simulink model "DVVMPTC_motor"  (R2021a)
settings: Solver=VariableStepAuto  StartTime=0.0  StopTime=10.0  RelTol=1e-3
libraries: powerlib_extras x3, spsDCVoltageSourceLib x2, spsPermanentMagnetSynchronousMachineLib x2, spsUniversalBridgeLib x2, spsVoltageMeasurementLib x2, spspowerguiLib x2, pid_lib x1, simulink x1
settings Model: Creator=86188  LastModifiedBy=86188

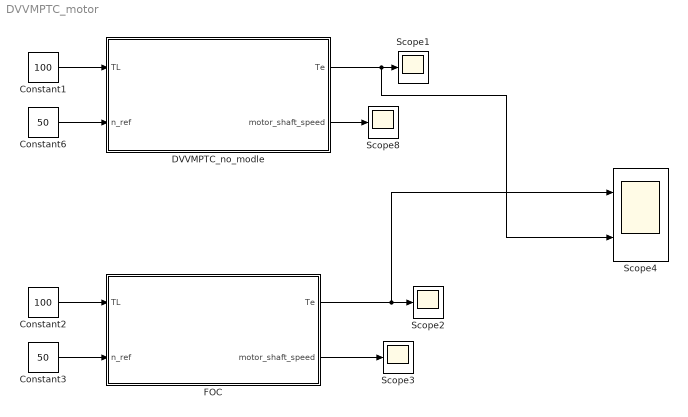
== system DVVMPTC_motor ==
  Constant1 : Constant  Value=100
  Constant2 : Constant  Value=100
  Constant3 : Constant  Value=50
  Constant6 : Constant  Value=50
  DVVMPTC_no_modle : Subsystem
  FOC : Subsystem
  Scope{1..3,8} (4 alike) : Scope
  Scope4 : Scope  NumInputPorts=2
  wires:
  DVVMPTC_no_modle/2(motor_shaft_speed) -> Scope8/1
  Constant1/1 -> DVVMPTC_no_modle/1(TL)
  Constant6/1 -> DVVMPTC_no_modle/2(n_ref)
  DVVMPTC_no_modle/1(Te) -> Scope4/2, Scope1/1
  Constant2/1 -> FOC/1(TL)
  Constant3/1 -> FOC/2(n_ref)
  FOC/1(Te) -> Scope4/1, Scope2/1
  FOC/2(motor_shaft_speed) -> Scope3/1

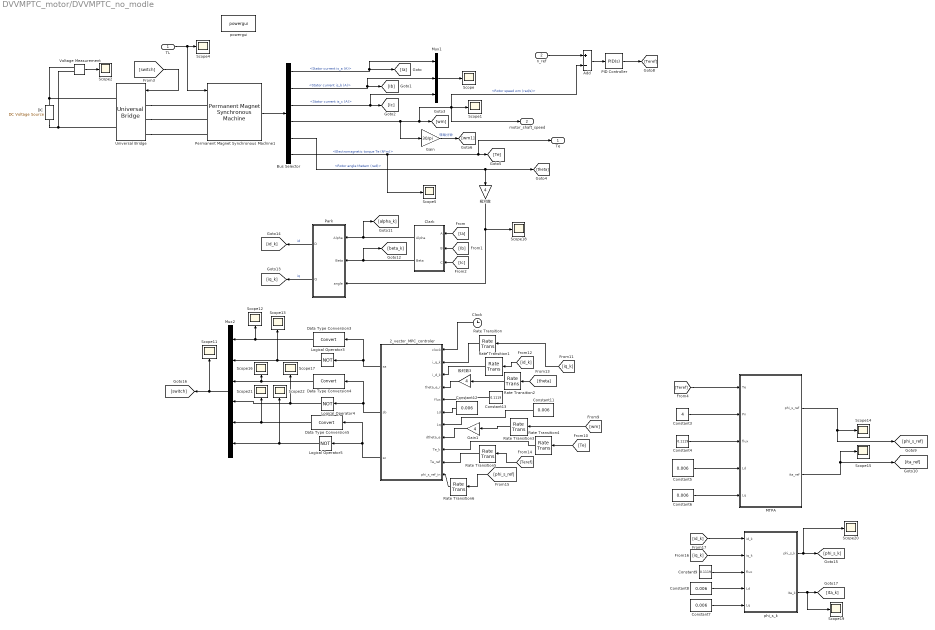
== system DVVMPTC_motor/DVVMPTC_no_modle ==
  TL : Inport
  n_ref : Inport  Port=2
  2_vector_MPC_controler : MATLAB Function  TreatAsAtomicUnit=on  SystemSampleTime=1e-5
  Add : Sum  Inputs=+-
  Bus Selector : BusSelector  OutputSignals=Stator current is_a (A),Stator current is_b (A),Stator current is_c (A),Rotor speed wm (rad/s),Rotor angle thetam (rad),Electromagnetic torque Te (N*m)
  Clark : Subsystem
  Clock : Clock
  Constant{5..8,11..12} (6 alike) : Constant  Value=0.006
  Constant13 : Constant  Value=0.1119
  Constant3 : Constant  Value=4
  Constant4 : Constant  Value=0.1119
  Constant9 : Constant  Value=0.1119
  DC : spsDCVoltageSourceLib/DC Voltage Source  Amplitude=400  Measurements=None
  Data Type Conversion3 : DataTypeConversion
  Data Type Conversion4 : DataTypeConversion
  Data Type Conversion5 : DataTypeConversion
  Gain : Gain  Gain=30/pi
  Gain1 : Gain  Gain=4
  Logical Operator3 : Logic  Operator=NOT  AllPortsSameDT=off  OutDataTypeStr=boolean
  Logical Operator4 : Logic  Operator=NOT  AllPortsSameDT=off  OutDataTypeStr=boolean
  Logical Operator5 : Logic  Operator=NOT  AllPortsSameDT=off  OutDataTypeStr=boolean
  MTPA : MATLAB Function  TreatAsAtomicUnit=on
  Mux1 : Mux  Inputs=3
  Mux2 : Mux  Inputs=6
  PID Controller : pid_lib/PID Controller  Controller=PID  Form=Parallel  TimeDomain=Continuous-time  UseExternalTs=off  SampleTime=-1  IntegratorMethod=Forward Euler  FilterMethod=Forward Euler  ControllerParametersSource=internal  P=5  I=1  D=0  UseFilter=on  N=100  TunerSelectOption=Transfer Function Based (PID Tuner App)  InitialConditionSource=internal  InitialConditionForIntegrator=0  InitialConditionForFilter=0  DifferentiatorICPrevScaledInput=0  ExternalReset=none  TrackingMode=off  Kt=1  LimitOutput=off  SatLimitsSource=internal  UpperSaturationLimit=inf  LowerSaturationLimit=-inf  LinearizeAsGain=on  AntiWindupMode=none  Kb=1  POutMin=[]  POutMax=[]  IOutMin=[]  IOutMax=[]  DOutMin=[]  DOutMax=[]  NOutMin=[]  NOutMax=[]  SumOutMin=[]  SumOutMax=[]  SaturationOutMin=[]  SaturationOutMax=[]  PParamMin=[]  PParamMax=[]  IParamMin=[]  IParamMax=[]  DParamMin=[]  DParamMax=[]  NParamMin=[]  NParamMax=[]  KbParamMin=[]  KbParamMax=[]  KtParamMin=[]  KtParamMax=[]  KbOutMin=[]  KbOutMax=[]  KtOutMin=[]  KtOutMax=[]  IntegratorOutMin=[]  IntegratorOutMax=[]  FilterOutMin=[]  FilterOutMax=[]  SumI1OutMin=[]  SumI1OutMax=[]  SumI2OutMin=[]  SumI2OutMax=[]  SumI3OutMin=[]  SumI3OutMax=[]  SumI4OutMin=[]  SumI4OutMax=[]  SumDOutMin=[]  SumDOutMax=[]  DifferentiatorOutMin=[]  DifferentiatorOutMax=[]  FilterDiffOutCoefMin=[]  FilterDiffOutCoefMax=[]  ReciprocalOutMin=[]  ReciprocalOutMax=[]  SumDenOutMin=[]  SumDenOutMax=[]  SumNumOutMin=[]  SumNumOutMax=[]  DivideOutMin=[]  DivideOutMax=[]  UdiffTsProdOutMin=[]  UdiffTsProdOutMax=[]  NTsProdOutMin=[]  NTsProdOutMax=[]  UintegralTsProdOutMin=[]  UintegralTsProdOutMax=[]  UngainTsProdOutMin=[]  UngainTsProdOutMax=[]  IntegratorContinuousStateAttributes=''  IntegratorStateMustResolveToSignalObject=off  IntegratorRTWStateStorageClass=Auto  FilterContinuousStateAttributes=''  FilterStateMustResolveToSignalObject=off  FilterRTWStateStorageClass=Auto  ParallelPVariant=InternalParameters  IdealPVariant=Disabled  IVariant=InternalParameters  DVariant=InternalParameters  IntegratorVariant=Continuous  SatVariant=Disabled  AWVariant=Passthrough  PCopyVariant=Disabled  TRVariant=Disabled  FdbkBlocksVariant=Forward  IdealPFdbkVariant=Disabled  SatFdbkVariant=Disabled  DerivativeFilterVariant=ContFilter  NVariant=InternalParameters  NCopyVariant=Disabled  FilterICVariant=InternalICsFilter  IntegratorICVariant=InternalICs  ExternalResetVariant=Disabled  TRSumVariant=Passthrough  SumFdbkVariant=Disabled  SumVariant=Sum_PID  TsampFilterVariant=InternalTs  TsampNgainVariant=Passthrough  TsampIntegralVariant=Passthrough  ExternalSaturationOutDataTypeStr=Inherit: Same as second input
  Park : Subsystem
  Permanent Magnet Synchronous Machine1 : spsPermanentMagnetSynchronousMachineLib/Permanent Magnet Synchronous Machine  NbPhases=3  FluxDistribution=Sinusoidal  RotorType=Salient-pole  MechanicalLoad=Torque Tm  PresetModel=No  ShowDetailedParameters=on  MeasurementBus=off  Resistance=0.11  Inductance=8.5e-3  dqInductances=[0.006 0.006]  La=0.000835  MachineConstant=Flux linkage established by magnets (V.s)  Flux=0.1119  VoltageCst=81.1857  TorqueCst=0.6714  Flat=120  Mechanical=[0.04 0.0002024 4 0]  PolePairs=4  InitialConditions=[0,0, 0,0]  InitialConditions5ph=[0 0 0 0 0 0]  RefAngle=Aligned with phase A axis (original Park)  IterativeDiscreteModel=Trapezoidal non iterative  TsBlock=-1  TsPowergui=0
  Rate Transition : RateTransition  OutPortSampleTime=1e-5
  Rate Transition1 : RateTransition  OutPortSampleTime=1e-5
  Rate Transition2 : RateTransition  OutPortSampleTime=1e-5
  Rate Transition{3..6} (4 alike) : RateTransition  OutPortSampleTime=1e-4
  Scope{,1..2,4..5,11..22} (17 alike) : Scope
  Universal Bridge : spsUniversalBridgeLib/Universal Bridge  Arms=3  SnubberResistance=1e5  SnubberCapacitance=inf  Device=IGBT / Diodes  Ron=1e-3  Lon=0  ForwardVoltages="[  0  0  ]"  ForwardVoltage=0  GTOparameters=[ 10e-6 , 20e-6 ]  IGBTparameters=[ 1e-6 , 2e-6 ]  Measurements=None  Measurements_2=None  converterType=Rectifier
  Voltage Measurement : spsVoltageMeasurementLib/Voltage Measurement  PhasorSimulation=off  OutputType=Complex  PSBequivalent=0
  phi_s_k : MATLAB Function  TreatAsAtomicUnit=on
  powergui : spspowerguiLib/powergui  Priority=1  SimulationMode=Discrete  SampleTime=1e-6  frequency=60  Iterations=50  frequencyindice=0  Pbase=100e6  ErrMax=1e-4  UnitsV=kV  UnitsW=MW  buscounter=0  FunctionMessages=off  echomessages=off  EnableUseOfTLC=off  CurrentSourceSwitches=off  DisableSnubberDevices=off  DisableRonSwitches=off  DisableVfSwitches=off  DisplayEquations=off  AutomaticDiscreteSolvers=off  SolverType=Tustin/Backward Euler (TBE)  Interpol=off  ExternalGateDelay=off  methode=off  Ts=100  x0status=blocks  SPID=on  SwTol=0  HookPort=off  NonlinearTolerance=1e-4  nMaxIteration=100  ContinueOnMaxIteration=off  RestoreLinks=warning  ResistiveCurrentMeasurement=off  Frange=[0:2:500]  Ylog=off  Xlog=on  ShowGrid=off  save=off  variable=ZData  structure=0  ZoomFFT=off  StartTime=0.0  cycles=1  DisplayStyle=1  fundamental=60  FreqAxis=off  MaxFrequency=1000  frequencyindicesteady=1  RmsSteady=1  display=off
  极对数 : Gain  Gain=4
  极对数3 : Gain  Gain=4
  Te : Outport
  motor_shaft_speed : Outport  Port=2
  wires:
  TL/1 -> Scope4/1, Permanent Magnet Synchronous Machine1/1
  Rate Transition6/1 -> 2_vector_MPC_controler/11(phi_s_ref_in)
  Rate Transition5/1 -> 2_vector_MPC_controler/10(Te_ref)
  Rate Transition4/1 -> 2_vector_MPC_controler/9(Te_k)
  Rate Transition3/1 -> Gain1/1
  Rate Transition2/1 -> 极对数3/1
  Rate Transition1/1 -> 2_vector_MPC_controler/3(i_d_k)
  Rate Transition/1 -> 2_vector_MPC_controler/2(i_q_k)
  phi_s_k/2(ita_k) -> [ita_k], Scope19/1
  极对数3/1 -> 2_vector_MPC_controler/4(theta_e_r)
  Mux2/1 -> [switch], Scope11/1
  Logical Operator5/1 -> Scope22/1, Mux2/6
  Data Type Conversion5/1 -> Scope21/1, Mux2/5
  Logical Operator4/1 -> Scope17/1, Mux2/4
  Data Type Conversion4/1 -> Scope16/1, Mux2/3
  Logical Operator3/1 -> Scope13/1, Mux2/2
  Data Type Conversion3/1 -> Scope12/1, Mux2/1
  2_vector_MPC_controler/3(sc) -> Logical Operator5/1, Data Type Conversion5/1
  2_vector_MPC_controler/2(sb) -> Logical Operator4/1, Data Type Conversion4/1
  2_vector_MPC_controler/1(sa) -> Logical Operator3/1, Data Type Conversion3/1
  [id_k] -> phi_s_k/1(id_k)
  [iq_k] -> phi_s_k/2(iq_k)
  phi_s_k/1(phi_s_k) -> Scope20/1, [phi_s_k]
  Constant9/1 -> phi_s_k/3(flux)
  Constant8/1 -> phi_s_k/4(Ld)
  Constant7/1 -> phi_s_k/5(Lq)
  MTPA/1(phi_s_ref) -> Scope14/1, [phi_s_ref]
  MTPA/2(ita_ref) -> [ita_ref], Scope15/1
  Constant6/1 -> MTPA/5(Lq)
  Constant5/1 -> MTPA/4(Ld)
  Constant4/1 -> MTPA/3(flux)
  Constant3/1 -> MTPA/2(Pn)
  [Teref] -> MTPA/1(Te)
  Clock/1 -> 2_vector_MPC_controler/1(clock)
  Permanent Magnet Synchronous Machine1/1 -> Bus Selector/1
  Bus Selector/1 -> Mux1/1, [Ia]  "<Stator current is_a (A)>"
  Bus Selector/2 -> Mux1/2, [Ib]  "<Stator current is_b (A)>"
  Bus Selector/3 -> Mux1/3, [Ic]  "<Stator current is_c (A)>"
  Bus Selector/4 -> Gain/1, motor_shaft_speed/1, Add/2, Scope1/1, [wm]  "<Rotor speed wm (rad/s)>"
  Bus Selector/5 -> 极对数/1, [theta]  "<Rotor angle thetam (rad)>"
  Bus Selector/6 -> [Te], Te/1, Scope5/1  "<Electromagnetic torque Te (N*m)>"
  Gain/1 -> [wm1]  "转每分钟"
  Clark/1(Alpha) -> Park/1(Alpha), [alpha_k]
  Clark/2(Beta) -> [beta_k], Park/2(Beta)
  [Ia] -> Clark/1(A)
  [Ib] -> Clark/2(B)
  [Ic] -> Clark/3(C)
  极对数/1 -> Park/3(angle), Scope18/1
  Park/1(D) -> [id_k]  "id"
  Park/2(Q) -> [iq_k]  "iq"
  [switch] -> Universal Bridge/1
  Mux1/1 -> Scope/1
  Gain1/1 -> 2_vector_MPC_controler/8(dtheta_e)
  Constant12/1 -> 2_vector_MPC_controler/6(Ld)
  Constant11/1 -> 2_vector_MPC_controler/7(Lq)
  Constant13/1 -> 2_vector_MPC_controler/5(flux)
  [Teref] -> Rate Transition5/1
  [phi_s_ref] -> Rate Transition6/1
  [iq_k] -> Rate Transition/1
  [id_k] -> Rate Transition1/1
  [theta] -> Rate Transition2/1
  [wm] -> Rate Transition3/1
  [Te] -> Rate Transition4/1
  n_ref/1 -> Add/1
  Voltage Measurement/1 -> Scope2/1
  PID Controller/1 -> [Teref]
  Add/1 -> PID Controller/1
  connections:
  Universal Bridge/LConn2 -- Permanent Magnet Synchronous Machine1/LConn2
  Universal Bridge/LConn3 -- Permanent Magnet Synchronous Machine1/LConn3
  DC/RConn1 -- Voltage Measurement/LConn1 -- Universal Bridge/RConn1
  DC/LConn1 -- Voltage Measurement/LConn2 -- Universal Bridge/RConn2
  Universal Bridge/LConn1 -- Permanent Magnet Synchronous Machine1/LConn1

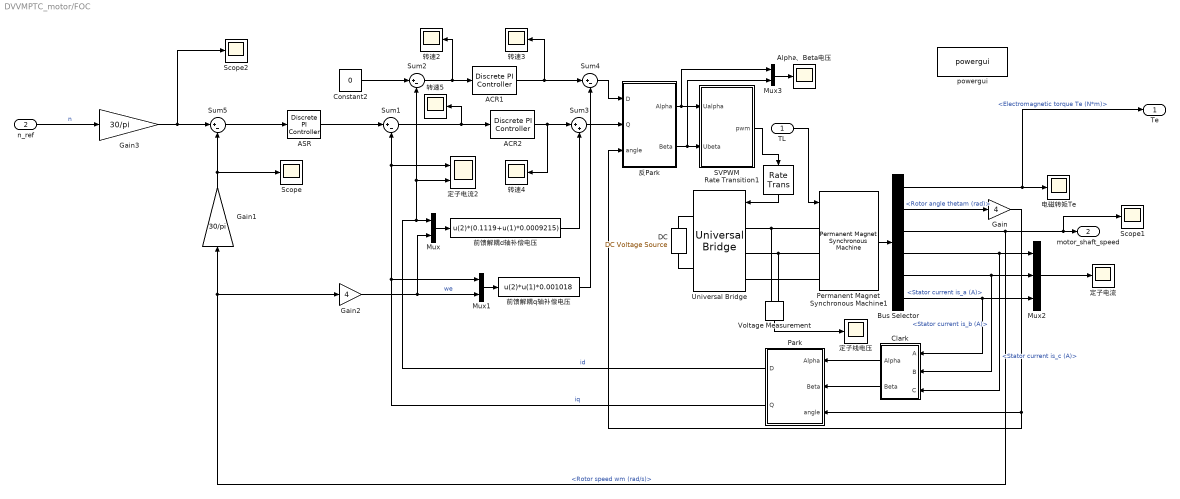
== system DVVMPTC_motor/FOC ==
  TL : Inport
  n_ref : Inport  Port=2
  ACR1 : powerlib_extras/Discrete  Control Blocks/Discrete PI Controller  Kp=4  Ki=80  Par_Limits=[760*0.9*sqrt(1/3) -760*0.9*sqrt(1/3)]  Init=0  Ts=1e-6
  ACR2 : powerlib_extras/Discrete  Control Blocks/Discrete PI Controller  Kp=4  Ki=80  Par_Limits=[760*0.9*sqrt(1/3) -760*0.9*sqrt(1/3)]  Init=0  Ts=1e-6
  ASR : powerlib_extras/Discrete  Control Blocks/Discrete PI Controller  Kp=0.8  Ki=10  Par_Limits=[1000 -1000]  Init=0  Ts=1e-6
  Alpha、Beta电压 : Scope
  Bus Selector : BusSelector  OutputSignals=Electromagnetic torque Te (N*m),Rotor angle thetam (rad),Rotor speed wm (rad/s),Stator current is_c (A),Stator current is_b (A),Stator current is_a (A)
  Clark : Subsystem
  Constant2 : Constant  Value=0
  DC : spsDCVoltageSourceLib/DC Voltage Source  Amplitude=560  Measurements=None
  Gain : Gain  Gain=4
  Gain1 : Gain  Gain=30/pi
  Gain2 : Gain  Gain=4
  Gain3 : Gain  Gain=30/pi
  Mux : Mux  Inputs=2
  Mux1 : Mux  Inputs=2
  Mux2 : Mux  Inputs=3
  Mux3 : Mux  Inputs=2
  Park : Subsystem
  Permanent Magnet Synchronous Machine1 : spsPermanentMagnetSynchronousMachineLib/Permanent Magnet Synchronous Machine  NbPhases=3  FluxDistribution=Sinusoidal  RotorType=Salient-pole  MechanicalLoad=Torque Tm  PresetModel=No  ShowDetailedParameters=on  MeasurementBus=off  Resistance=0.11  Inductance=8.5e-3  dqInductances=[0.006 0.006]  La=0.000835  MachineConstant=Flux linkage established by magnets (V.s)  Flux=0.1119  VoltageCst=81.1857  TorqueCst=0.6714  Flat=120  Mechanical=[0.04 0.0002024 4 0]  PolePairs=4  InitialConditions=[0,0, 0,0]  InitialConditions5ph=[0 0 0 0 0 0]  RefAngle=Aligned with phase A axis (original Park)  IterativeDiscreteModel=Trapezoidal non iterative  TsBlock=-1  TsPowergui=0
  Rate Transition1 : RateTransition  OutPortSampleTime=1e-5
  SVPWM : Subsystem
  Scope : Scope
  Scope1 : Scope
  Scope2 : Scope
  Sum{1..2,4..5} (4 alike) : Sum  Inputs=|+-
  Sum3 : Sum  Inputs=|++
  Universal Bridge : spsUniversalBridgeLib/Universal Bridge  Arms=3  SnubberResistance=1e5  SnubberCapacitance=inf  Device=IGBT / Diodes  Ron=1e-3  Lon=0  ForwardVoltages="[  0  0  ]"  ForwardVoltage=0  GTOparameters=[ 10e-6 , 20e-6 ]  IGBTparameters=[ 1e-6 , 2e-6 ]  Measurements=None  Measurements_2=None  converterType=Rectifier
  Voltage Measurement : spsVoltageMeasurementLib/Voltage Measurement  PhasorSimulation=off  OutputType=Complex  PSBequivalent=0
  powergui : spspowerguiLib/powergui  Priority=1  SimulationMode=Discrete  SampleTime=1e-6  frequency=60  Iterations=50  frequencyindice=0  Pbase=100e6  ErrMax=1e-4  UnitsV=kV  UnitsW=MW  buscounter=0  FunctionMessages=off  echomessages=off  EnableUseOfTLC=off  CurrentSourceSwitches=off  DisableSnubberDevices=off  DisableRonSwitches=off  DisableVfSwitches=off  DisplayEquations=off  AutomaticDiscreteSolvers=off  SolverType=Tustin  Interpol=off  ExternalGateDelay=off  methode=off  Ts=0  x0status=blocks  SPID=off  SwTol=0  HookPort=off  NonlinearTolerance=1e-4  nMaxIteration=100  ContinueOnMaxIteration=off  RestoreLinks=warning  ResistiveCurrentMeasurement=off  Frange=[0:2:500]  Ylog=off  Xlog=on  ShowGrid=off  save=off  variable=ZData  structure=ScopeData7  ZoomFFT=on  StartTime=2.5  cycles=3  DisplayStyle=1  fundamental=60  FreqAxis=off  MaxFrequency=2000  frequencyindicesteady=1  RmsSteady=1  display=off
  前馈解耦d轴补偿电压 : Fcn  Expr=u(2)*(0.1119+u(1)*0.0009215)
  前馈解耦q轴补偿电压 : Fcn  Expr=u(2)*u(1)*0.001018
  反Park : Subsystem
  定子电流 : Scope
  定子电流2 : Scope  NumInputPorts=2
  定子线电压 : Scope
  电磁转矩Te : Scope
  转速{2..5} (4 alike) : Scope
  Te : Outport
  motor_shaft_speed : Outport  Port=2
  wires:
  Gain3/1 -> Sum5/1, Scope2/1
  Gain1/1 -> Scope/1, Sum5/2
  ASR/1 -> Sum1/1
  Voltage Measurement/1 -> 定子线电压/1
  前馈解耦q轴补偿电压/1 -> Sum4/2
  Sum2/1 -> ACR1/1, 转速2/1
  Mux2/1 -> 定子电流/1
  Bus Selector/6 -> Clark/1(A), Mux2/3  "<Stator current is_a (A)>"
  Sum5/1 -> ASR/1
  Clark/1(Alpha) -> Park/1(Alpha)
  Permanent Magnet Synchronous Machine1/1 -> Bus Selector/1
  Park/2(Q) -> Sum1/2, 定子电流2/1, Mux1/1  "iq"
  Clark/2(Beta) -> Park/2(Beta)
  Sum1/1 -> ACR2/1, 转速5/1
  Mux3/1 -> Alpha、Beta电压/1
  反Park/1(Alpha) -> SVPWM/1(Ualpha), Mux3/1
  Bus Selector/3 -> motor_shaft_speed/1, Scope1/1, Gain1/1, Gain2/1  "<Rotor speed wm (rad/s)>"
  Mux/1 -> 前馈解耦d轴补偿电压/1
  反Park/2(Beta) -> SVPWM/2(Ubeta), Mux3/2
  Sum3/1 -> 反Park/2(Q)
  Park/1(D) -> Mux/1, Sum2/2, 定子电流2/2  "id"
  Bus Selector/1 -> 电磁转矩Te/1, Te/1  "<Electromagnetic torque Te (N*m)>"
  Bus Selector/5 -> Clark/2(B), Mux2/2  "<Stator current is_b (A)>"
  Bus Selector/2 -> Gain/1  "<Rotor angle thetam (rad)>"
  n_ref/1 -> Gain3/1  "n"
  前馈解耦d轴补偿电压/1 -> Sum3/2
  ACR2/1 -> Sum3/1, 转速4/1
  Sum4/1 -> 反Park/1(D)
  SVPWM/1(pwm) -> Rate Transition1/1
  Mux1/1 -> 前馈解耦q轴补偿电压/1
  Gain2/1 -> Mux/2, Mux1/2  "we"
  Gain/1 -> Park/3(angle), 反Park/3(angle)
  Constant2/1 -> Sum2/1
  Bus Selector/4 -> Clark/3(C), Mux2/1  "<Stator current is_c (A)>"
  ACR1/1 -> Sum4/1, 转速3/1
  TL/1 -> Permanent Magnet Synchronous Machine1/1
  Rate Transition1/1 -> Universal Bridge/1
  connections:
  Voltage Measurement/LConn1 -- Permanent Magnet Synchronous Machine1/LConn1 -- Universal Bridge/LConn1
  Voltage Measurement/LConn2 -- Permanent Magnet Synchronous Machine1/LConn2 -- Universal Bridge/LConn2
  DC/RConn1 -- Universal Bridge/RConn1
  Permanent Magnet Synchronous Machine1/LConn3 -- Universal Bridge/LConn3
  DC/LConn1 -- Universal Bridge/RConn2

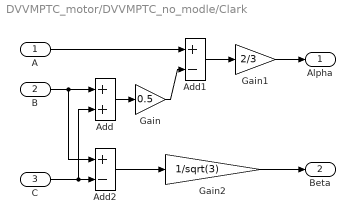
== system DVVMPTC_motor/DVVMPTC_no_modle/Clark ==
  A : Inport
  B : Inport  Port=2
  C : Inport  Port=3
  Add : Sum
  Add1 : Sum  Inputs=+-
  Add2 : Sum  Inputs=+-
  Gain : Gain  Gain=0.5
  Gain1 : Gain  Gain=2/3
  Gain2 : Gain  Gain=1/sqrt(3)
  Alpha : Outport
  Beta : Outport  Port=2
  wires:
  B/1 -> Add2/1, Add/1
  C/1 -> Add/2, Add2/2
  Add/1 -> Gain/1
  A/1 -> Add1/1
  Gain/1 -> Add1/2
  Add1/1 -> Gain1/1
  Gain1/1 -> Alpha/1
  Add2/1 -> Gain2/1
  Gain2/1 -> Beta/1

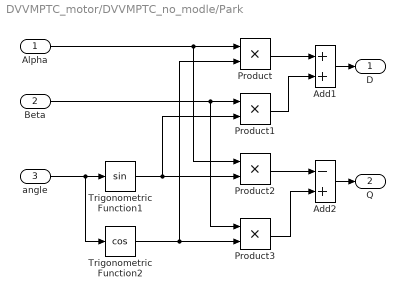
== system DVVMPTC_motor/DVVMPTC_no_modle/Park ==
  Alpha : Inport
  Beta : Inport  Port=2
  angle : Inport  Port=3
  Add1 : Sum
  Add2 : Sum  Inputs=-+
  Product{,1..3} (4 alike) : Product
  Trigonometric Function1 : Trigonometry
  Trigonometric Function2 : Trigonometry  Operator=cos
  D : Outport
  Q : Outport  Port=2
  wires:
  Add2/1 -> Q/1
  Product3/1 -> Add2/2
  Product2/1 -> Add2/1
  Add1/1 -> D/1
  Product1/1 -> Add1/2
  Product/1 -> Add1/1
  Trigonometric Function1/1 -> Product2/2, Product1/2
  Beta/1 -> Product3/1, Product1/1
  Trigonometric Function2/1 -> Product3/2, Product/2
  Alpha/1 -> Product2/1, Product/1
  angle/1 -> Trigonometric Function1/1, Trigonometric Function2/1

== system DVVMPTC_motor/FOC/Clark ==
  A : Inport
  B : Inport  Port=2
  C : Inport  Port=3
  Add : Sum
  Add1 : Sum  Inputs=+-
  Add2 : Sum  Inputs=+-
  Gain : Gain  Gain=0.5
  Gain1 : Gain  Gain=2/3
  Gain2 : Gain  Gain=1/sqrt(3)
  Alpha : Outport
  Beta : Outport  Port=2
  wires:
  Gain2/1 -> Beta/1
  Add2/1 -> Gain2/1
  Gain1/1 -> Alpha/1
  Add1/1 -> Gain1/1
  Gain/1 -> Add1/2
  A/1 -> Add1/1
  Add/1 -> Gain/1
  C/1 -> Add2/2, Add/2
  B/1 -> Add/1, Add2/1

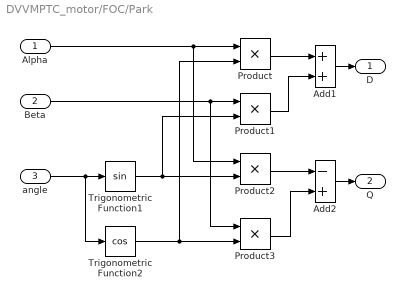
== system DVVMPTC_motor/FOC/Park ==
  Alpha : Inport
  Beta : Inport  Port=2
  angle : Inport  Port=3
  Add1 : Sum
  Add2 : Sum  Inputs=-+
  Product{,1..3} (4 alike) : Product
  Trigonometric Function1 : Trigonometry
  Trigonometric Function2 : Trigonometry  Operator=cos
  D : Outport
  Q : Outport  Port=2
  wires:
  angle/1 -> Trigonometric Function2/1, Trigonometric Function1/1
  Alpha/1 -> Product/1, Product2/1
  Trigonometric Function2/1 -> Product/2, Product3/2
  Beta/1 -> Product1/1, Product3/1
  Trigonometric Function1/1 -> Product1/2, Product2/2
  Product/1 -> Add1/1
  Product1/1 -> Add1/2
  Add1/1 -> D/1
  Product2/1 -> Add2/1
  Product3/1 -> Add2/2
  Add2/1 -> Q/1

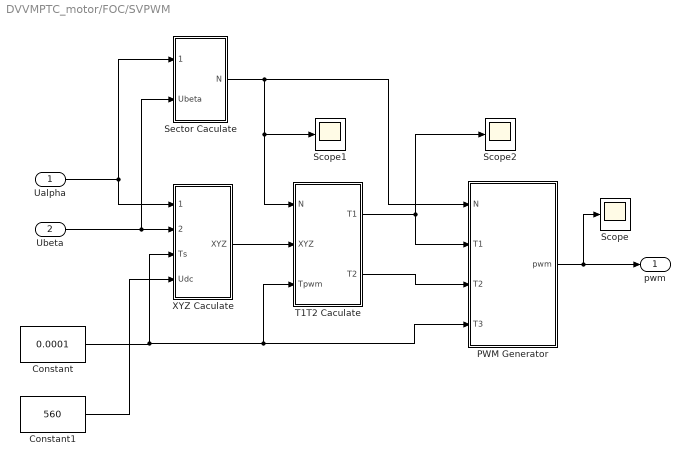
== system DVVMPTC_motor/FOC/SVPWM ==
  Ualpha : Inport
  Ubeta : Inport  Port=2
  Constant : Constant  Value=0.0001
  Constant1 : Constant  Value=560
  PWM Generator : Subsystem
  Scope : Scope
  Scope1 : Scope
  Scope2 : Scope
  Sector Caculate : Subsystem
  T1T2 Caculate : Subsystem
  XYZ Caculate : Subsystem
  pwm : Outport
  wires:
  PWM Generator/1(pwm) -> Scope/1, pwm/1
  T1T2 Caculate/2(T2) -> PWM Generator/3(T2)
  T1T2 Caculate/1("T1 ") -> Scope2/1, PWM Generator/2(T1)
  Sector Caculate/1(N) -> PWM Generator/1(N), T1T2 Caculate/1(N), Scope1/1
  XYZ Caculate/1(XYZ) -> T1T2 Caculate/2(XYZ)
  Constant1/1 -> XYZ Caculate/4(Udc)
  Constant/1 -> XYZ Caculate/3(Ts), T1T2 Caculate/3(Tpwm), PWM Generator/4(T3)
  Ubeta/1 -> XYZ Caculate/2(Ubeta), Sector Caculate/2("Ubeta ")
  Ualpha/1 -> Sector Caculate/1(Ualpha), XYZ Caculate/1(Ualpha)

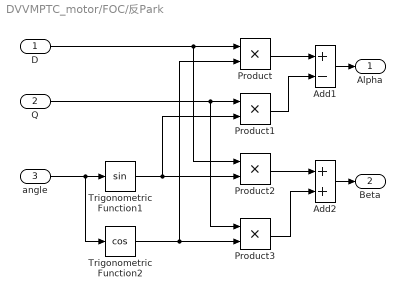
== system DVVMPTC_motor/FOC/反Park ==
  D : Inport
  Q : Inport  Port=2
  angle : Inport  Port=3
  Add1 : Sum  Inputs=+-
  Add2 : Sum
  Product{,1..3} (4 alike) : Product
  Trigonometric Function1 : Trigonometry
  Trigonometric Function2 : Trigonometry  Operator=cos
  Alpha : Outport
  Beta : Outport  Port=2
  wires:
  Add2/1 -> Beta/1
  Product3/1 -> Add2/2
  Product2/1 -> Add2/1
  Add1/1 -> Alpha/1
  Product1/1 -> Add1/2
  Product/1 -> Add1/1
  Trigonometric Function1/1 -> Product2/2, Product1/2
  Q/1 -> Product3/1, Product1/1
  Trigonometric Function2/1 -> Product3/2, Product/2
  D/1 -> Product2/1, Product/1
  angle/1 -> Trigonometric Function1/1, Trigonometric Function2/1

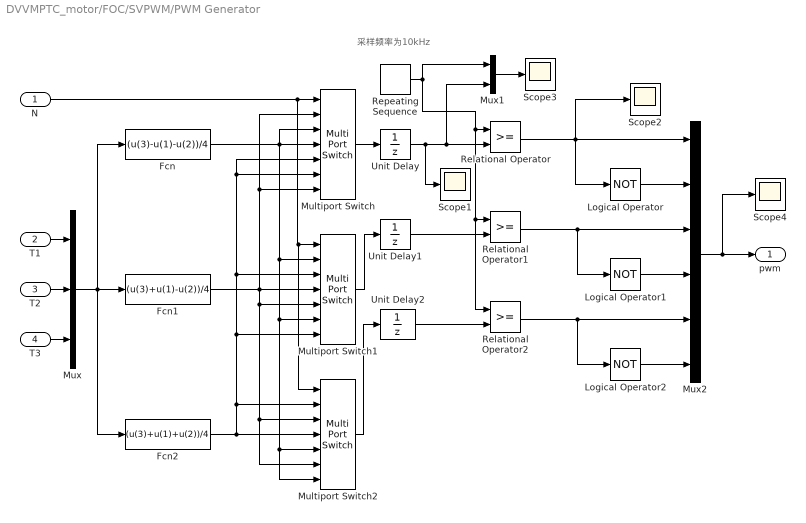
== system DVVMPTC_motor/FOC/SVPWM/PWM Generator ==
  note: 采样频率为10kHz
  N : Inport
  T1 : Inport  Port=2
  T2 : Inport  Port=3
  T3 : Inport  Port=4
  Fcn : Fcn  Expr=(u(3)-u(1)-u(2))/4
  Fcn1 : Fcn  Expr=(u(3)+u(1)-u(2))/4
  Fcn2 : Fcn  Expr=(u(3)+u(1)+u(2))/4
  Logical Operator : Logic  Operator=NOT  AllPortsSameDT=off  OutDataTypeStr=boolean
  Logical Operator1 : Logic  Operator=NOT  AllPortsSameDT=off  OutDataTypeStr=boolean
  Logical Operator2 : Logic  Operator=NOT  AllPortsSameDT=off  OutDataTypeStr=boolean
  Multiport Switch : MultiPortSwitch  Inputs=6  DiagnosticForDefault=None
  Multiport Switch1 : MultiPortSwitch  Inputs=6  DiagnosticForDefault=None
  Multiport Switch2 : MultiPortSwitch  Inputs=6  DiagnosticForDefault=None
  Mux : Mux  Inputs=3
  Mux1 : Mux  Inputs=2
  Mux2 : Mux  Inputs=6
  Relational Operator : RelationalOperator  OutDataTypeStr=boolean  RndMeth=Nearest
  Relational Operator1 : RelationalOperator  OutDataTypeStr=boolean  RndMeth=Nearest
  Relational Operator2 : RelationalOperator  OutDataTypeStr=boolean  RndMeth=Nearest
  Repeating Sequence : simulink/Sources/Repeating Sequence  rep_seq_t=[0 0.00005 0.0001]  rep_seq_y=[0 0.00005 0]
  Scope{1..4} (4 alike) : Scope
  Unit Delay : UnitDelay  SampleTime=0.0001  HasFrameUpgradeWarning=on
  Unit Delay1 : UnitDelay  SampleTime=0.0001  HasFrameUpgradeWarning=on
  Unit Delay2 : UnitDelay  SampleTime=0.0001  HasFrameUpgradeWarning=on
  pwm : Outport
  wires:
  Unit Delay2/1 -> Relational Operator2/2
  Unit Delay1/1 -> Relational Operator1/2
  Unit Delay/1 -> Scope1/1, Relational Operator/2, Mux1/2
  Mux1/1 -> Scope3/1
  Multiport Switch/1 -> Unit Delay/1
  Multiport Switch2/1 -> Unit Delay2/1
  Multiport Switch1/1 -> Unit Delay1/1
  Mux2/1 -> pwm/1, Scope4/1
  Logical Operator2/1 -> Mux2/6
  Logical Operator1/1 -> Mux2/4
  Logical Operator/1 -> Mux2/2
  Relational Operator2/1 -> Mux2/5, Logical Operator2/1
  Relational Operator1/1 -> Mux2/3, Logical Operator1/1
  Relational Operator/1 -> Mux2/1, Logical Operator/1, Scope2/1
  Repeating Sequence/1 -> Relational Operator/1, Relational Operator1/1, Relational Operator2/1, Mux1/1
  Fcn2/1 -> Multiport Switch/5, Multiport Switch/6, Multiport Switch1/3, Multiport Switch1/7, Multiport Switch2/2, Multiport Switch2/4
  Fcn1/1 -> Multiport Switch1/4, Multiport Switch1/5, Multiport Switch2/3, Multiport Switch2/6, Multiport Switch/2, Multiport Switch/7
  Fcn/1 -> Multiport Switch/3, Multiport Switch/4, Multiport Switch1/2, Multiport Switch1/6, Multiport Switch2/5, Multiport Switch2/7
  N/1 -> Multiport Switch/1, Multiport Switch1/1, Multiport Switch2/1
  Mux/1 -> Fcn2/1, Fcn1/1, Fcn/1
  T3/1 -> Mux/3
  T1/1 -> Mux/1
  T2/1 -> Mux/2

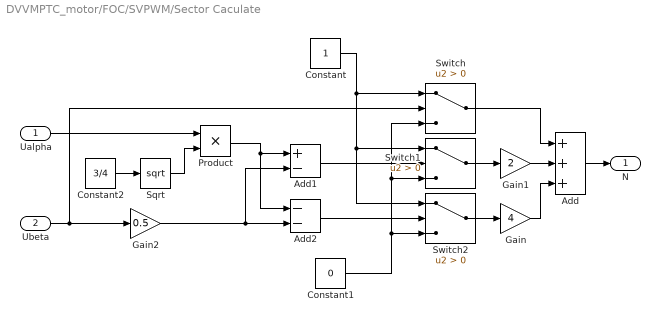
== system DVVMPTC_motor/FOC/SVPWM/Sector Caculate ==
  Ualpha : Inport
  "Ubeta " : Inport  Port=2
  Add : Sum  Inputs=+++
  Add1 : Sum  Inputs=+-
  Add2 : Sum  Inputs=--
  Constant : Constant
  Constant1 : Constant  Value=0
  Constant2 : Constant  Value=3/4
  Gain : Gain  Gain=4
  Gain1 : Gain  Gain=2
  Gain2 : Gain  Gain=0.5
  Product : Product
  Sqrt : Sqrt  SaturateOnIntegerOverflow=on
  Switch : Switch  Criteria=u2 > Threshold
  Switch1 : Switch  Criteria=u2 > Threshold
  Switch2 : Switch  Criteria=u2 > Threshold
  N : Outport
  wires:
  Gain2/1 -> Add2/2, Add1/2
  Product/1 -> Add1/1, Add2/1
  Sqrt/1 -> Product/2
  Constant2/1 -> Sqrt/1
  Switch/1 -> Add/1
  Switch1/1 -> Gain1/1
  Switch2/1 -> Gain/1
  Gain/1 -> Add/3
  Gain1/1 -> Add/2
  Add/1 -> N/1
  Constant1/1 -> Switch/3, Switch1/3, Switch2/3
  Constant/1 -> Switch2/1, Switch1/1, Switch/1
  Add2/1 -> Switch2/2
  Add1/1 -> Switch1/2
  "Ubeta "/1 -> Gain2/1, Switch/2
  Ualpha/1 -> Product/1

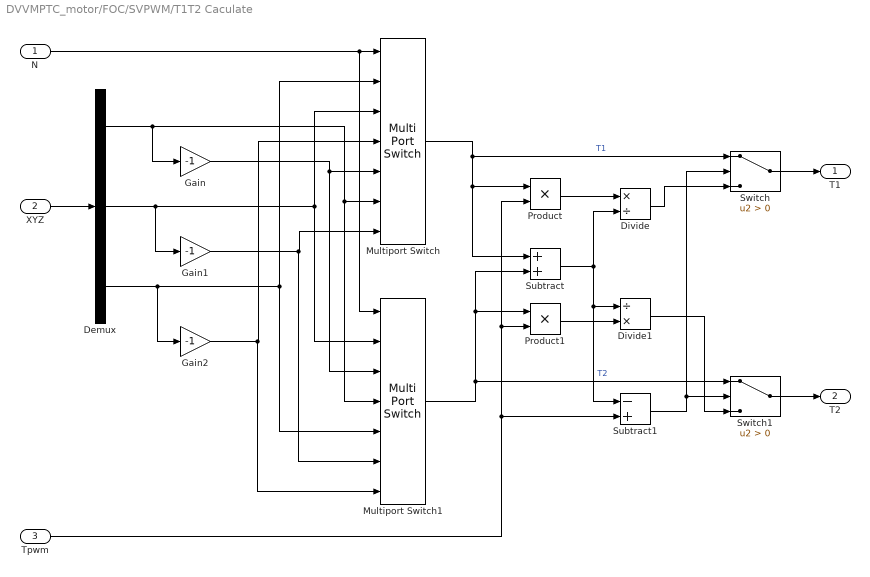
== system DVVMPTC_motor/FOC/SVPWM/T1T2 Caculate ==
  N : Inport
  XYZ : Inport  Port=2
  Tpwm : Inport  Port=3
  Demux : Demux  Outputs=3
  Divide : Product  Inputs=*/
  Divide1 : Product  Inputs=/*
  Gain : Gain  Gain=-1
  Gain1 : Gain  Gain=-1
  Gain2 : Gain  Gain=-1
  Multiport Switch : MultiPortSwitch  Inputs=6  DiagnosticForDefault=None
  Multiport Switch1 : MultiPortSwitch  Inputs=6  DiagnosticForDefault=None
  Product : Product
  Product1 : Product
  Subtract : Sum
  Subtract1 : Sum  Inputs=-+
  Switch : Switch  Criteria=u2 > Threshold
  Switch1 : Switch  Criteria=u2 > Threshold
  "T1 " : Outport
  T2 : Outport  Port=2
  wires:
  Product1/1 -> Divide1/2
  Subtract/1 -> Subtract1/1, Divide1/1, Divide/2
  Product/1 -> Divide/1
  Switch/1 -> "T1 "/1
  Switch1/1 -> T2/1
  Subtract1/1 -> Switch/2, Switch1/2
  Divide1/1 -> Switch1/3
  Divide/1 -> Switch/3
  Tpwm/1 -> Product1/2, Product/2, Subtract1/2
  Multiport Switch1/1 -> Switch1/1, Product1/1, Subtract/2  "T2"
  Multiport Switch/1 -> Subtract/1, Product/1, Switch/1  "T1"
  XYZ/1 -> Demux/1
  Gain2/1 -> Multiport Switch/4, Multiport Switch1/7
  Gain1/1 -> Multiport Switch/7, Multiport Switch1/6
  Gain/1 -> Multiport Switch1/3, Multiport Switch/5
  Demux/3 -> Multiport Switch/2, Multiport Switch1/5, Gain2/1
  Demux/2 -> Gain1/1, Multiport Switch1/2, Multiport Switch/3
  Demux/1 -> Gain/1, Multiport Switch/6, Multiport Switch1/4
  N/1 -> Multiport Switch/1, Multiport Switch1/1

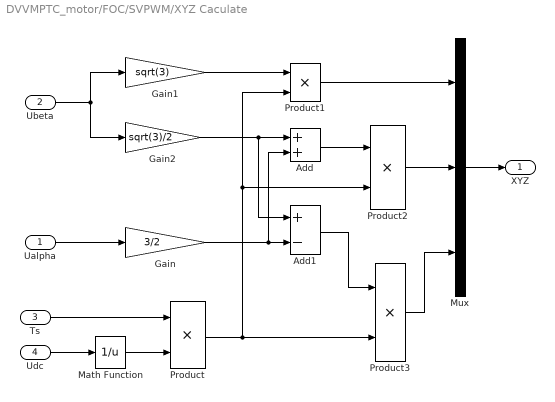
== system DVVMPTC_motor/FOC/SVPWM/XYZ Caculate ==
  Ualpha : Inport
  Ubeta : Inport  Port=2
  Ts : Inport  Port=3
  Udc : Inport  Port=4
  Add : Sum
  Add1 : Sum  Inputs=+-
  Gain : Gain  Gain=3/2
  Gain1 : Gain  Gain=sqrt(3)
  Gain2 : Gain  Gain=sqrt(3)/2
  Math Function : Math  Operator=reciprocal  SignedPower=on  SaturateOnIntegerOverflow=on
  Mux : Mux  Inputs=3
  Product{,1..3} (4 alike) : Product
  XYZ : Outport
  wires:
  Mux/1 -> XYZ/1
  Product2/1 -> Mux/2
  Add1/1 -> Product3/1
  Add/1 -> Product2/1
  Gain2/1 -> Add/1, Add1/1
  Gain/1 -> Add1/2, Add/2
  Product3/1 -> Mux/3
  Product/1 -> Product3/2, Product2/2, Product1/2
  Product1/1 -> Mux/1
  Gain1/1 -> Product1/1
  Math Function/1 -> Product/2
  Udc/1 -> Math Function/1
  Ts/1 -> Product/1
  Ubeta/1 -> Gain1/1, Gain2/1
  Ualpha/1 -> Gain/1

== matlab function DVVMPTC_motor/DVVMPTC_no_modle/2_vector_MPC_controler ==
  settings: updateMethod=DISCRETE
  data: clock input; i_q_k input; i_d_k input; theta_e_r input; sa output; sb output; sc output; flux input; Ld input; Lq input; dtheta_e input; Te_k input; Te_ref input; phi_s_ref_in input
function [sa, sb, sc] = fcn(clock, i_q_k, i_d_k, theta_e_r, flux, Ld, Lq, dtheta_e, Te_k, Te_ref, phi_s_ref_in)
    %% 0. 参数初始化
    Ts = 0.0001;     % 控制周期 100us
    vdc = 400;       % 母线电压
    Rs = 0.11;       % 定子电阻
    pn = 4;          % 极对数
    
    %% 1. 状态预测（一拍延时补偿） - 核心修复点
    % 论文公式 (5) 或 (6)。此处使用前向欧拉法预测 k+1 时刻的电流
    % 注意：此时假定 k 时刻施加的电压是上一个周期计算出的最优电压
    % 但在 Simulink 仿真中，通常需要将上个周期的 u_opt 反馈回来。
    % 如果没有反馈，可以用近似方法：假设当前电流已经包含了一部分过去的影响，
    % 但更标准的做法是预测。这里简化处理，基于当前电流和反电势预测下一刻的趋势。
    
    % 在实际 MPTC 中，必须利用 k 时刻的 u(k) 来预测 i(k+1)
    % 这里为了简化，我们至少要补偿旋转导致的相位角变化
    theta_e_k1 = theta_e_r + dtheta_e * Ts; 
    
    % 使用论文公式(5)进行电流预测 (需要上个周期的电压，这里暂用反电势模型近似补偿相位)
    % 严谨做法：Function 增加输入 u_alpha_old, u_beta_old
    % 这里采用论文中忽略电阻压降后的磁链预测公式(7)的简化逻辑：
    
    % 计算 k 时刻的磁链
    phi_d_k = Ld * i_d_k + flux;
    phi_q_k = Lq * i_q_k;
    
    % 预测 k+1 时刻的磁链 (基于旋转坐标系，假设稳态时 d/dt=0，主要变化由旋转引起)
    % 论文公式 (7) 的核心思想
    phi_d_k1 = phi_d_k + (dtheta_e * phi_q_k) * Ts; 
    phi_q_k1 = phi_q_k - (dtheta_e * phi_d_k) * Ts;
    
    % 更新预测后的电流 (用于后续计算)
    % i_d_k1 = (phi_d_k1 - flux) / Ld; % 如果是 IPMSM
    % i_q_k1 = phi_q_k1 / Lq;
    
    % 为了解决"掉落到负载转矩"的问题，必须修正用于计算参考电压的磁链值
    % 使用预测值代替测量值
    phi_d_calc = phi_d_k1;
    phi_q_calc = phi_q_k1;
    
    %% 2. 磁链参考值修正 - 核心修复点
    % 死拍控制要求非常严格，如果 Te_ref 很大，导致需要的 iq 很大，
    % 此时总磁链 sqrt(phid^2 + phiq^2) 必然增加。
    % 如果输入的 phi_s_ref 太小（例如只给 flux），方程无解，导致转矩上不去。
    % 这里根据 MTPA (id=0) 原则动态计算最小所需磁链
    
    % 基于 MTPA (id=0) 计算期望的 q 轴磁链
    expected_iq = Te_ref / (1.5 * pn * flux); 
    expected_phi_q = Lq * expected_iq;
    expected_phi_d = flux; % id=0 时
    
    % 计算物理上兼容的磁链参考值
    min_phi_s = sqrt(expected_phi_d^2 + expected_phi_q^2);
    
    % 如果输入的参考值小于物理限制，则覆盖它
    if phi_s_ref_in < min_phi_s
        phi_s_ref = min_phi_s;
    else
        phi_s_ref = phi_s_ref_in;
    end

    %% 3. DB-DTFC 计算参考电压 (基于预测的 k+1 状态计算 k+2 的需求)
    % 论文公式 (12) 和相关系数
    % X1 对应 d 轴电压方程中的耦合项
    X1 = phi_d_calc + dtheta_e * phi_q_calc * Ts;
    
    % B 对应 q 轴电压方程中的项 (包含转矩误差反馈)
    % 注意：这里用 Te_ref - Te_k，如果 Te_k 滞后，这里增益会很大。
    % 理想情况下应使用预测转矩 Te_k1，但使用 Te_k 在低速下尚可。
    B = ((2*Lq)/(3*pn*flux))*(Te_ref - Te_k) + (Rs*Ts*phi_q_calc)/Lq + dtheta_e*Ts*phi_d_calc;
    
    % 求解 d 轴电压 (二次方程)
    % (X1 + ud*Ts)^2 + (B)^2 = phi_s_ref^2
    % 展开：X1^2 + 2*X1*ud*Ts + ud^2*Ts^2 + B^2 = phi_s_ref^2
    % 整理为标准形式 a*x^2 + b*x + c = 0
    % a = Ts^2
    % b = 2*X1*Ts
    % c = X1^2 + B^2 - phi_s_ref^2
    
    % 你原本的代码逻辑似乎来源于论文的另一种推导，但这里直接用勾股定理推导更直观且等价
    % 你的代码 X2 计算有点复杂，这里简化逻辑以确保数值稳定
    
    term_c = X1^2 + B^2 - phi_s_ref^2;
    delta = (2*X1*Ts)^2 - 4 * (Ts^2) * term_c;
    
    if delta < 0
        delta = 0; % 强行有解，防止复数
    end
    
    % 求解 ud
    ud_sol1 = (-2*X1*Ts + sqrt(delta)) / (2*Ts^2);
    ud_sol2 = (-2*X1*Ts - sqrt(delta)) / (2*Ts^2);
    
    % 选择绝对值较小的电压矢量（能量最小原理）
    if abs(ud_sol1) < abs(ud_sol2)
        ud_ref = ud_sol1;
    else
        ud_ref = ud_sol2;
    end
    
    uq_ref = B / Ts;

    %% 4. 坐标变换 (dq -> alpha/beta)
    % 注意：必须使用 k+1 时刻的角度进行变换，因为电压是在 k+1 时刻发出的
    u_alpha_ref = cos(theta_e_k1)*ud_ref - sin(theta_e_k1)*uq_ref;
    u_beta_ref  = sin(theta_e_k1)*ud_ref + cos(theta_e_k1)*uq_ref;
    
    theta_u_ref = atan2(u_beta_ref, u_alpha_ref);
    if theta_u_ref < 0
        theta_u_ref = theta_u_ref + 2*pi;
    end

    %% 5. 第一扇区及矢量选择
    theta_norm_rel = theta_u_ref + pi/6; % 偏移30度以匹配扇区定义
    if theta_norm_rel > 2*pi
        theta_norm_rel = theta_norm_rel - 2*pi;
    end

    sector = floor(theta_norm_rel / (pi/3)) + 1;
    if sector > 6 
        sector = 1; % 修正 sector=7 的情况
    end
    
    % 电压矢量定义 (0-7)
    % 对应: V0, V1(100), V2(110), V3(010), V4(011), V5(001), V6(101), V7
    voltage_vectors = [
        0 0 0; % 0 (Index 1)
        1 0 0; % 1 (Index 2)
        1 1 0; % 2 (Index 3)
        0 1 0; % 3 (Index 4)
        0 1 1; % 4 (Index 5)
        0 0 1; % 5 (Index 6)
        1 0 1; % 6 (Index 7)
        1 1 1];% 7 (Index 8)

    first_vector_idx = sector + 1; 
    first_vector = voltage_vectors(first_vector_idx, :);

    %% 6. 第二矢量选择 (MPTC-II: 遍历相邻矢量)
    % 将 Alpha-Beta 坐标系下的 8 个基础电压矢量预先计算出来
    v_basic_alpha = zeros(8,1);
    v_basic_beta = zeros(8,1);
    const_k = 2/3 * vdc;
    for k = 1:8
        sa_t = voltage_vectors(k,1); sb_t = voltage_vectors(k,2); sc_t = voltage_vectors(k,3);
        u_an = vdc/3 * (2*sa_t - sb_t - sc_t);
        u_bn = vdc/3 * (2*sb_t - sa_t - sc_t);
        u_cn = vdc/3 * (2*sc_t - sa_t - sb_t); % 仅用于推导
        v_basic_alpha(k) = u_an;
        v_basic_beta(k)  = u_bn/sqrt(3); % 注意变换系数
        % 你的代码里用的是: 2/3*(sqrt(3)/2*u_bn - sqrt(3)/2*u_cn) = 1/sqrt(3)*(u_bn-u_cn)
        % 标准Clarke: beta = 1/sqrt(3)*(2ub - ub - uc)? 不，标准是 (2*ub - ua - uc)?
        % 你的变换: u_alpha = 2/3(u_an - 0.5u_bn - 0.5u_cn) -> 正确
        % 你的变换: u_beta = 2/3(sqrt(3)/2 * u_bn - sqrt(3)/2 * u_cn) -> 正确
    end
    
    % 定义相邻扇区索引 (注意 MATLAB 索引从 1 开始)
    % V1(idx2) neighbors: V2(idx3), V6(idx7), V0(idx1), V7(idx8)
    adjacent_indices = {
        [3, 7, 1, 8]; % Sector 1 (V1) -> V2, V6, V0, V7
        [2, 4, 1, 8]; % Sector 2 (V2) -> V1, V3, ...
        [3, 5, 1, 8]; % Sector 3 (V3)
        [4, 6, 1, 8]; % Sector 4 (V4)
        [5, 7, 1, 8]; % Sector 5 (V5)
        [6, 2, 1, 8]  % Sector 6 (V6)
    };
    
    candidates = adjacent_indices{sector};
    min_cost = inf;
    second_vector_idx = candidates(1);
    
    % 你的 Cost Function: J = |u_ref - u_second|
    % 论文 Cost Function: J = |u_ref - t1*u1 - t2*u2|
    % 这里你使用的是 MPTC-II 的简化版选择策略（基于位置），这是可以的
    % 但更准确的是像论文 Eq(25) 那样把时间代入后计算，这里保留你的逻辑以最小化变动
    
    for idx = candidates
        cost = sqrt((u_alpha_ref - v_basic_alpha(idx))^2 + (u_beta_ref - v_basic_beta(idx))^2);
        if cost < min_cost
            min_cost = cost;
            second_vector_idx = idx;
        end
    end
    second_vector = voltage_vectors(second_vector_idx, :);

    %% 7. 矢量作用时间计算
    u1_a = v_basic_alpha(first_vector_idx);
    u1_b = v_basic_beta(first_vector_idx);
    u2_a = v_basic_alpha(second_vector_idx);
    u2_b = v_basic_beta(second_vector_idx);
    
    % 投影法计算占空比 d1 (即 t_1opt / Ts)
    % u_ref = d1 * u1 + (1-d1) * u2
    % u_ref - u2 = d1 * (u1 - u2)
    % d1 = dot(u_ref - u2, u1 - u2) / |u1 - u2|^2
    
    vec_diff_a = u1_a - u2_a;
    vec_diff_b = u1_b - u2_b;
    denominator = vec_diff_a^2 + vec_diff_b^2;
    
    if denominator < 1e-6
        % 如果两个矢量相同（例如都是零矢量），时间分配无意义，全给1
        d1 = 1;
    else
        numerator = (u_alpha_ref - u2_a) * vec_diff_a + (u_beta_ref - u2_b) * vec_diff_b;
        d1 = numerator / denominator;
    end
    
    % 饱和限制
    if d1 > 1; d1 = 1; end
    if d1 < 0; d1 = 0; end
    
    t_1opt = d1 * Ts;

    %% 8. PWM 输出
    % 需要一个静态变量记录当前周期起始时间，你原来的代码写得没问题
    % 但为了防止 clock 溢出或步长问题，建议直接用 Simulink 的 Digital Clock 模块输入
    % 这里假设 clock 是当前仿真时间
    
    persistent t_cycle_start
    if isempty(t_cycle_start)
        t_cycle_start = 0;
    end
    
    % 简单的 PWM 逻辑
    % 在一个周期内，前 t_1opt 时间发 first_vector，剩下时间发 second_vector
    
    % 计算当前周期内的相对时间
    relative_t = mod(clock, Ts);
    
    if relative_t < t_1opt
        sa = first_vector(1);
        sb = first_vector(2);
        sc = first_vector(3);
    else
        sa = second_vector(1);
        sb = second_vector(2);
        sc = second_vector(3);
    end
end

== matlab function DVVMPTC_motor/DVVMPTC_no_modle/MTPA ==
  data: Te input; phi_s_ref output; Pn input; flux input; Ld input; Lq input; ita_ref output
function [phi_s_ref, ita_ref] = fcn(Te, Pn, flux, Ld, Lq)
%% MPTA原则计算phi_s_ref和ita_ref
% 对于表贴式PMSM (Ld = Lq)，MPTA条件就是id=0控制

% 计算q轴电流参考（id_ref = 0）
iq_ref = Te / (1.5 * Pn * flux);

% 计算定子磁链参考值
% phi_d = flux + Ld * id_ref = flux
% phi_q = Lq * iq_ref
phi_d_ref = flux;      % id=0
phi_q_ref = Lq * iq_ref;

phi_s_ref = sqrt(phi_d_ref^2 + phi_q_ref^2);

% 计算定子磁链参考角度
if abs(Te) < 1e-6
    ita_ref = 0;  % 零转矩时角度为0
else
    ita_ref = atan2(phi_q_ref, phi_d_ref);
end

% 确保角度在合理范围内
ita_ref = real(ita_ref);  % 避免复数
end

== matlab function DVVMPTC_motor/DVVMPTC_no_modle/phi_s_k ==
  data: id_k input; phi_s_k output; iq_k input; flux input; Ld input; Lq input; ita_k output
function [phi_s_k,ita_k]  = fcn(id_k,iq_k,flux,Ld,Lq)
phi_q_k = Lq*iq_k;
phi_d_k = Ld*id_k + flux;
phi_s_k = sqrt(phi_q_k^2+phi_d_k^2);
ita_k = atan2(phi_q_k, phi_d_k);

end
